simulink model "e6"  (R2024b)
settings: Solver=VariableStepAuto  StartTime=0.0  StopTime=30  RelTol=1e-3
libraries: simulink x1
settings Model: Creator=Lenovo  LastModifiedBy=Lenovo

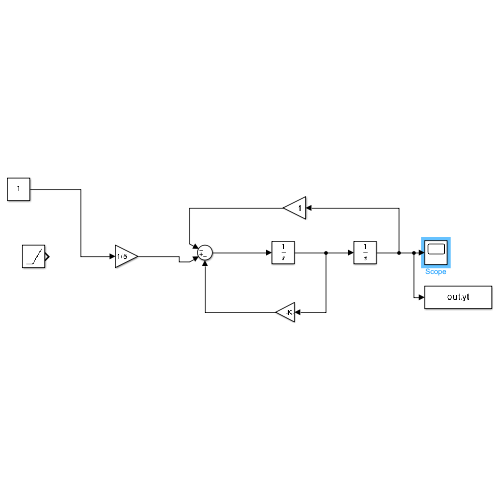
[thumbnail: Simulink's stored preview of the top-level diagram]
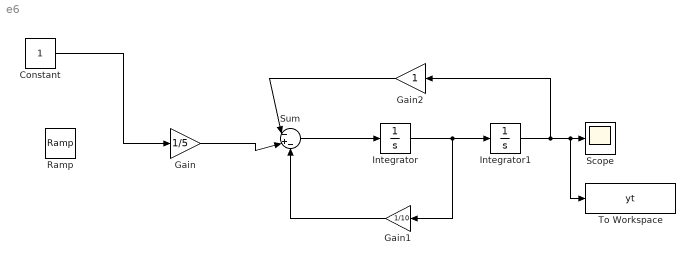
== system e6 ==
  Constant : Constant
  Gain : Gain  Gain=1/5
  Gain1 : Gain  Gain=1/10
  Gain2 : Gain
  Integrator : Integrator
  Integrator1 : Integrator
  Ramp : simulink/Sources/Ramp  slope=1  start=0  InitialOutput=0
  Scope : Scope
  Sum : Sum  Inputs=|-+-
  To Workspace : ToWorkspace  VariableName=yt  SaveFormat=Timeseries  SampleTime=-1
  wires:
  Gain1/1 -> Sum/3
  Integrator/1 -> Gain1/1, Integrator1/1
  Sum/1 -> Integrator/1
  Integrator1/1 -> Gain2/1, To Workspace/1, Scope/1
  Gain/1 -> Sum/2
  Gain2/1 -> Sum/1
  Constant/1 -> Gain/1
